simulink model "NonLinModelMracScaled"  (R2023b)
settings: Solver=ode4  StartTime=0.0  StopTime=50  FixedStep=1e-3  RelTol=1e-3
values from neighbouring files (symbols this model uses):
  Am_bar = A_bar - B_bar_mA * Km    [placePoles.m]
  B_bar_mA = B_bar .* 1e-3    [newDesign.m]
  Bm_bar_mm = B_bar_mA / DC_gain    [placePoles.m]
  Gamma_L = 1e-6    (= 1e-06)    [newDesign.m]
  Gamma_R = 1e-4    (= 0.0001)    [newDesign.m]
  L_hat_IC = -Km    [newDesign.m]
  M_hat_IC = 1 / DC_gain    [newDesign.m]
  P_bar = lyap(Am_bar', Q_bar)    [newDesign.m]
  P_return = 4.46e5    (= 446000)    [newDesign.m]
  PA_IC = PA_Pa.Data(1)    [newDesign.m]
  PB_IC = PB_Pa.Data(1)    [newDesign.m]
  Ps_supply = 199.85e5    (= 19985000)    [newDesign.m]
  sigma_L = 0.001    [newDesign.m]
  sigma_M = 0.001    [newDesign.m]
  xc_dot_IC = v_mPs.Data(1)    [newDesign.m]
  xc_IC = xc_m.Data(1)    [newDesign.m]
undefined symbols (not defined in the file or in its folder): AEFF, B_E, C_T, k, K, M, m3PsToLpm, PA_Pa, PB_Pa, r_v_mPs, V01, V02, V_DEAD, xc_m
settings Model: Creator=snr  LastModifiedBy=snr

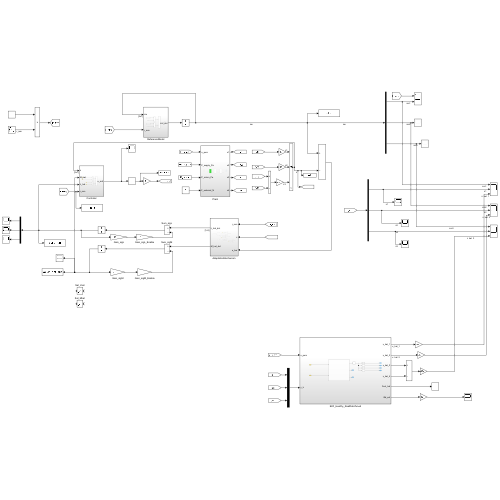
[thumbnail: Simulink's stored preview of the top-level diagram]
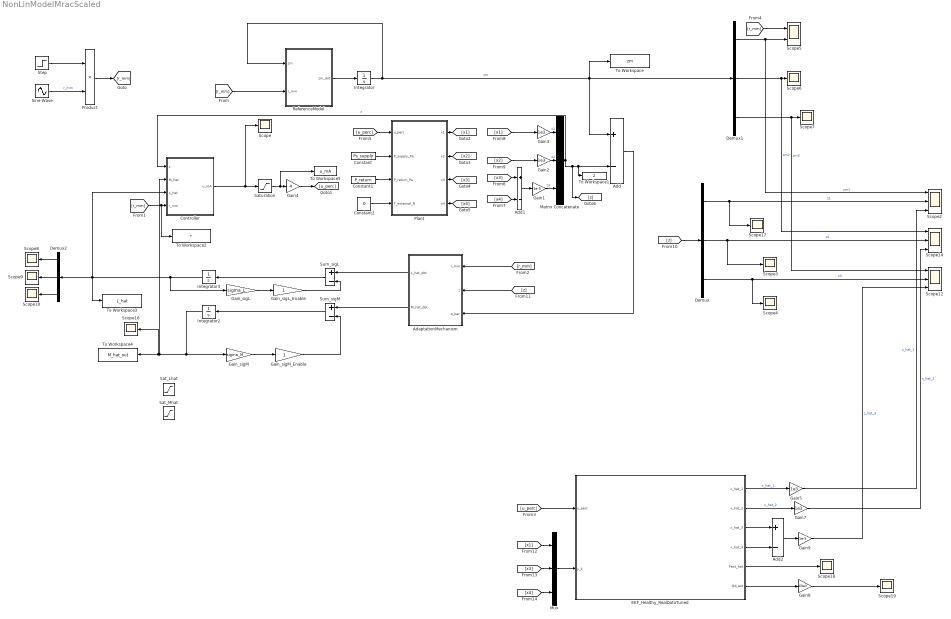
== system NonLinModelMracScaled ==
  AdaptationMechanism : Subsystem
  Add : Sum  Inputs=+-
  Add1 : Sum  Inputs=+-
  Add2 : Sum  Inputs=+-
  Constant : Constant  Value=Ps_supply
  Constant1 : Constant  Value=P_return
  Constant2 : Constant  Value=0
  Controller : Subsystem
  Demux : Demux  Outputs=3
  Demux1 : Demux  Outputs=3
  Demux2 : Demux  Outputs=3
  EKF_Healthy_RealDataTuned : Subsystem
  Gain1 : Gain  Gain=1e-5
  Gain{2..3,5,7} (4 alike) : Gain  Gain=1e3
  Gain4 : Gain  Gain=4
  Gain8 : Gain  Gain=60e3
  Gain9 : Gain  Gain=1e-5
  Gain_sigL : Gain  Gain=sigma_L
  Gain_sigL_Enable : Gain
  Gain_sigM : Gain  Gain=sigma_M
  Gain_sigM_Enable : Gain
  Integrator : Integrator  InitialCondition=[0;0;0]
  Integrator2 : Integrator  InitialCondition=M_hat_IC
  Integrator3 : Integrator  InitialCondition=L_hat_IC
  Matrix Concatenate : Concatenate  NumInputs=3  Mode=Multidimensional array
  Mux : Mux  Inputs=3
  Plant : Subsystem
  Product : Product
  ReferenceModel : Subsystem
  Sat_Lhat : Saturate  UpperLimit=0.125  LowerLimit=-0.125
  Sat_Mhat : Saturate  UpperLimit=0.12  LowerLimit=-0.12
  Saturation : Saturate  UpperLimit=25  LowerLimit=-25
  Scope{,3..4,6..10,16..19} (12 alike) : Scope
  Scope12 : Scope  NumInputPorts=3
  Scope14 : Scope  NumInputPorts=3
  Scope2 : Scope  NumInputPorts=3
  Scope5 : Scope  NumInputPorts=2
  Sine Wave : Sin  Amplitude=15  Frequency=2*pi*0.5  SampleTime=0
  Step : Step  Time=0  SampleTime=0
  Sum_sigL : Sum  Inputs=+-
  Sum_sigM : Sum  Inputs=+-
  To Workspace : ToWorkspace  VariableName=zm  SaveFormat=Timeseries  SampleTime=-1
  To Workspace1 : ToWorkspace  VariableName=z  SaveFormat=Timeseries  SampleTime=-1
  To Workspace2 : ToWorkspace  VariableName=r  SaveFormat=Timeseries  SampleTime=-1
  To Workspace3 : ToWorkspace  VariableName=L_hat  SaveFormat=Timeseries  SampleTime=-1
  To Workspace4 : ToWorkspace  VariableName=M_hat_out  SaveFormat=Timeseries  SampleTime=-1
  To Workspace5 : ToWorkspace  VariableName=u_mA  SaveFormat=Timeseries  SampleTime=-1
  wires:
  Constant2/1 -> Plant/4(F_external_N)
  Constant1/1 -> Plant/3(P_return_Pa)
  Gain1/1 -> Matrix Concatenate/3  "z3"
  Add1/1 -> Gain1/1
  Demux/2 -> Scope3/1, Scope14/2  "z2"
  Demux2/1 -> Scope8/1
  Demux2/3 -> Scope10/1
  [r_mm] -> ReferenceModel/2(r_mm)
  Demux2/2 -> Scope9/1
  Demux/3 -> Scope4/1, Scope12/2  "z3"
  [r_mm] -> AdaptationMechanism/1(r_mm)
  Sine Wave/1 -> Product/2  "r_mm"
  Demux1/1 -> Scope2/1, Scope5/2  "zm1"
  Demux1/2 -> Scope14/1, Scope6/1  "zm2"
  Integrator/1 -> To Workspace/1, Add/1, Demux1/1, ReferenceModel/1(zm)  "zm"
  Add/1 -> AdaptationMechanism/3(e_bar)
  Controller/1(u_mA) -> Scope/1, Saturation/1
  Demux1/3 -> Scope12/1, Scope7/1  "zm3"
  Demux/1 -> Scope17/1, Scope2/2  "z1"
  Constant/1 -> Plant/2(P_supply_Pa)
  Matrix Concatenate/1 -> [z], To Workspace1/1, Add/2, Controller/1(z)  "z"
  [r_mm] -> To Workspace2/1, Controller/4(r_mm)
  [r_mm] -> Scope5/1
  ReferenceModel/1(zm_dot) -> Integrator/1
  Gain2/1 -> Matrix Concatenate/2  "z2"
  Gain3/1 -> Matrix Concatenate/1  "z1"
  Saturation/1 -> To Workspace5/1, Gain4/1
  AdaptationMechanism/1(L_hat_dot) -> Sum_sigL/1
  Sum_sigL/1 -> Integrator3/1
  AdaptationMechanism/2(M_hat_dot) -> Sum_sigM/1
  Sum_sigM/1 -> Integrator2/1
  Step/1 -> Product/1
  Product/1 -> [r_mm]
  Mux/1 -> EKF_Healthy_RealDataTuned/2(y_k)
  EKF_Healthy_RealDataTuned/1(x_hat_1) -> Gain5/1  "x_hat_1"
  Gain5/1 -> Scope2/3  "z_hat_1"
  Gain4/1 -> [u_perc]
  EKF_Healthy_RealDataTuned/2(x_hat_2) -> Gain7/1  "x_hat_2"
  Gain7/1 -> Scope14/3  "z_hat_2"
  EKF_Healthy_RealDataTuned/5(Fext_hat) -> Scope18/1
  EKF_Healthy_RealDataTuned/6(Qd_est) -> Gain8/1
  Gain8/1 -> Scope19/1
  EKF_Healthy_RealDataTuned/4(x_hat_4) -> Add2/2
  EKF_Healthy_RealDataTuned/3(x_hat_3) -> Add2/1
  Add2/1 -> Gain9/1
  Gain9/1 -> Scope12/3  "z_hat_3"
  Integrator3/1 -> Gain_sigL/1, Demux2/1, To Workspace3/1, Controller/3(L_hat)
  Integrator2/1 -> Controller/2(M_hat), Scope16/1, To Workspace4/1, Gain_sigM/1
  Gain_sigM/1 -> Gain_sigM_Enable/1
  Gain_sigL/1 -> Gain_sigL_Enable/1
  Gain_sigM_Enable/1 -> Sum_sigM/2
  Gain_sigL_Enable/1 -> Sum_sigL/2
  [u_perc] -> EKF_Healthy_RealDataTuned/1(u_perc)
  [u_perc] -> Plant/1(u_perc)
  Plant/1(x1) -> [x1]
  Plant/2(x2) -> [x2]
  Plant/3(x3) -> [x3]
  Plant/4(x4) -> [x4]
  [x3] -> Add1/1
  [x4] -> Add1/2
  [x1] -> Gain3/1
  [x2] -> Gain2/1
  [z] -> Demux/1
  [z] -> AdaptationMechanism/2(z)
  [x1] -> Mux/1
  [x3] -> Mux/2
  [x4] -> Mux/3

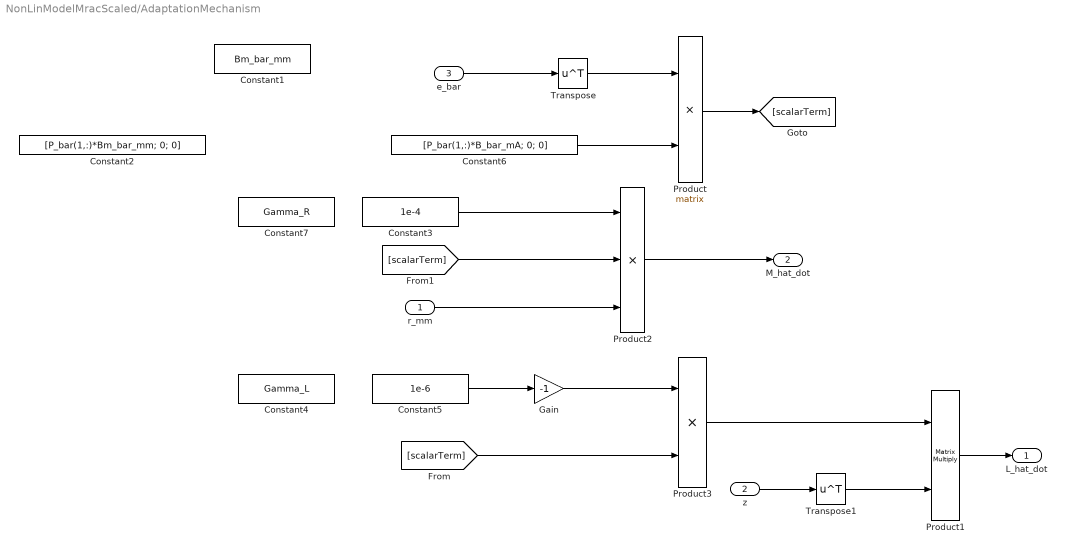
== system NonLinModelMracScaled/AdaptationMechanism ==
  r_mm : Inport
  z : Inport  Port=2
  e_bar : Inport  Port=3
  Constant1 : Constant  Value=Bm_bar_mm
  Constant2 : Constant  Value=[P_bar(1,:)*Bm_bar_mm; 0; 0]
  Constant3 : Constant  Value=1e-4
  Constant4 : Constant  Value=Gamma_L
  Constant5 : Constant  Value=1e-6
  Constant6 : Constant  Value=[P_bar(1,:)*B_bar_mA; 0; 0]
  Constant7 : Constant  Value=Gamma_R
  Gain : Gain  Gain=-1
  Product : Product  Multiplication=Matrix(*)
  Product1 : Product  Multiplication=Matrix(*)
  Product2 : Product  Inputs=3
  Product3 : Product
  Transpose : Math  Operator=transpose
  Transpose1 : Math  Operator=transpose
  L_hat_dot : Outport  PortDimensions=[1,3]
  M_hat_dot : Outport  Port=2
  wires:
  Gain/1 -> Product3/1
  Constant5/1 -> Gain/1
  Product1/1 -> L_hat_dot/1
  Transpose/1 -> Product/1
  Constant6/1 -> Product/2
  Product/1 -> [scalarTerm]
  [scalarTerm] -> Product3/2
  z/1 -> Transpose1/1
  Transpose1/1 -> Product1/2
  Product2/1 -> M_hat_dot/1
  Constant3/1 -> Product2/1
  [scalarTerm] -> Product2/2
  r_mm/1 -> Product2/3
  Product3/1 -> Product1/1
  e_bar/1 -> Transpose/1

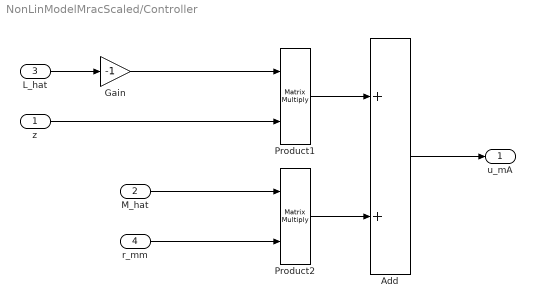
== system NonLinModelMracScaled/Controller ==
  z : Inport  PortDimensions=[3,1]
  M_hat : Inport  Port=2
  L_hat : Inport  Port=3
  r_mm : Inport  Port=4
  Add : Sum
  Gain : Gain  Gain=-1
  Product1 : Product  Multiplication=Matrix(*)
  Product2 : Product  Multiplication=Matrix(*)
  u_mA : Outport  PortDimensions=[1,1]
  wires:
  Add/1 -> u_mA/1
  Product1/1 -> Add/1
  Product2/1 -> Add/2
  L_hat/1 -> Gain/1
  z/1 -> Product1/2
  Gain/1 -> Product1/1
  M_hat/1 -> Product2/1
  r_mm/1 -> Product2/2

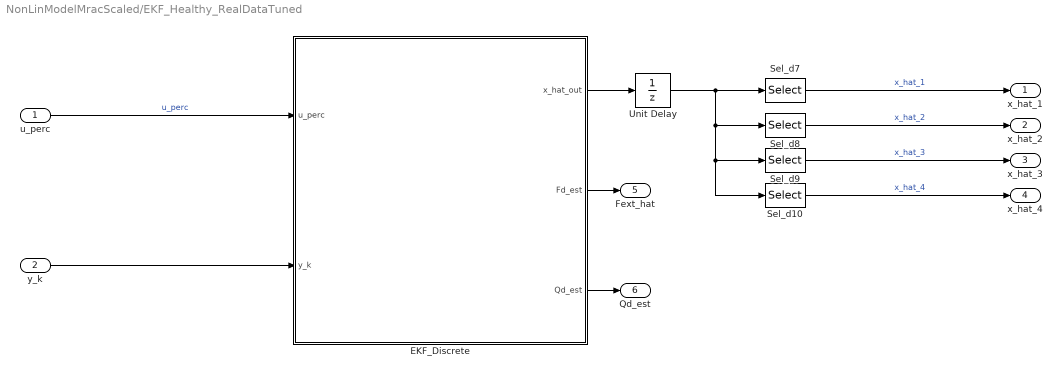
== system NonLinModelMracScaled/EKF_Healthy_RealDataTuned ==
  u_perc : Inport  OutDataTypeStr=double
  y_k : Inport  Port=2  OutDataTypeStr=double
  EKF_Discrete : MATLAB Function  TreatAsAtomicUnit=on  SystemSampleTime=1e-3
  Sel_d10 : Selector  InputPortWidth=6  IndexOptions=Index vector (dialog)  Indices=4  OutputSizes=1
  Sel_d7 : Selector  InputPortWidth=6  IndexOptions=Index vector (dialog)  Indices=1  OutputSizes=1
  Sel_d8 : Selector  InputPortWidth=6  IndexOptions=Index vector (dialog)  Indices=2  OutputSizes=1  RuntimeRangeChecks=on
  Sel_d9 : Selector  InputPortWidth=6  IndexOptions=Index vector (dialog)  Indices=3  OutputSizes=1
  Unit Delay : UnitDelay  InitialCondition=[xc_m.Data(1); r_v_mPs.Data(1); PA_Pa.Data(1); PB_Pa.Data(1); 0; 0]  SampleTime=1e-3  HasFrameUpgradeWarning=on
  x_hat_1 : Outport  OutDataTypeStr=double
  x_hat_2 : Outport  Port=2  OutDataTypeStr=double
  x_hat_3 : Outport  Port=3  OutDataTypeStr=double
  x_hat_4 : Outport  Port=4  OutDataTypeStr=double
  Fext_hat : Outport  Port=5  OutDataTypeStr=double
  Qd_est : Outport  Port=6  OutDataTypeStr=double
  wires:
  u_perc/1 -> EKF_Discrete/1(u_perc)  "u_perc"
  y_k/1 -> EKF_Discrete/2(y_k)
  EKF_Discrete/1(x_hat_out) -> Unit Delay/1
  Sel_d7/1 -> x_hat_1/1  "x_hat_1"
  Sel_d8/1 -> x_hat_2/1  "x_hat_2"
  Sel_d9/1 -> x_hat_3/1  "x_hat_3"
  Sel_d10/1 -> x_hat_4/1  "x_hat_4"
  EKF_Discrete/2(Fd_est) -> Fext_hat/1
  EKF_Discrete/3(Qd_est) -> Qd_est/1
  Unit Delay/1 -> Sel_d7/1, Sel_d10/1, Sel_d9/1, Sel_d8/1

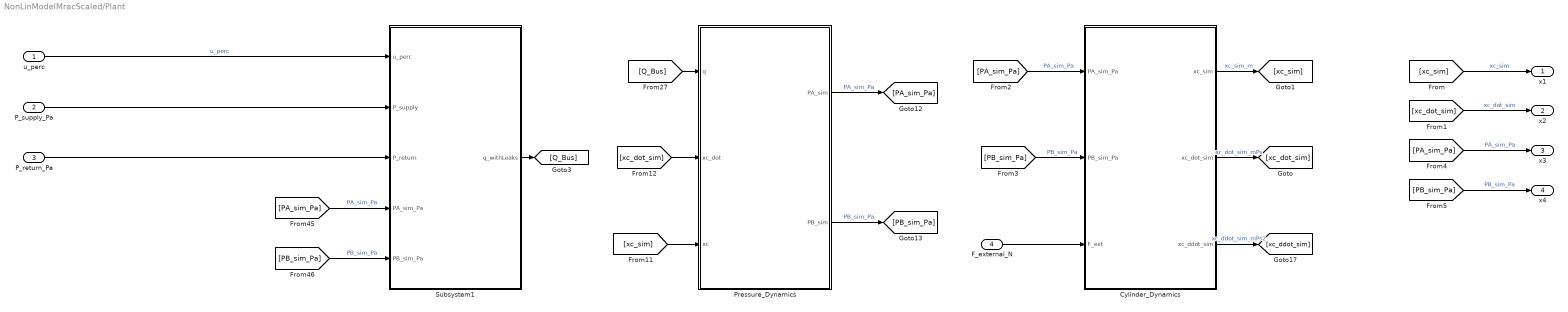
== system NonLinModelMracScaled/Plant ==
  u_perc : Inport  OutDataTypeStr=double
  P_supply_Pa : Inport  Port=2
  P_return_Pa : Inport  Port=3
  F_external_N : Inport  Port=4
  Cylinder_Dynamics : Subsystem
  Pressure_Dynamics : Subsystem
  Subsystem1 : Subsystem
  x1 : Outport
  x2 : Outport  Port=2
  x3 : Outport  Port=3
  x4 : Outport  Port=4
  wires:
  Cylinder_Dynamics/1(xc_sim) -> [xc_sim]  "xc_sim_m"
  [xc_sim] -> Pressure_Dynamics/3(xc)
  P_supply_Pa/1 -> Subsystem1/2(P_supply)
  [PA_sim_Pa] -> Subsystem1/4(PA_sim_Pa)  "PA_sim_Pa"
  [PB_sim_Pa] -> Subsystem1/5(PB_sim_Pa)  "PB_sim_Pa"
  [PB_sim_Pa] -> Cylinder_Dynamics/2(PB_sim_Pa)  "PB_sim_Pa"
  Pressure_Dynamics/1(PA_sim) -> [PA_sim_Pa]  "PA_sim_Pa"
  Cylinder_Dynamics/3(xc_ddot_sim) -> [xc_ddot_sim]  "xc_ddot_sim_mPs2"
  Cylinder_Dynamics/2(xc_dot_sim) -> [xc_dot_sim]  "xc_dot_sim_mPs"
  [xc_dot_sim] -> Pressure_Dynamics/2(xc_dot)
  [PA_sim_Pa] -> Cylinder_Dynamics/1(PA_sim_Pa)  "PA_sim_Pa"
  Pressure_Dynamics/2(PB_sim) -> [PB_sim_Pa]  "PB_sim_Pa"
  Subsystem1/1(q_withLeaks) -> [Q_Bus]
  [Q_Bus] -> Pressure_Dynamics/1(q)
  u_perc/1 -> Subsystem1/1(u_perc)  "u_perc"
  P_return_Pa/1 -> Subsystem1/3(P_return)
  F_external_N/1 -> Cylinder_Dynamics/3(F_ext)
  [xc_sim] -> x1/1  "xc_sim"
  [xc_dot_sim] -> x2/1  "xc_dot_sim"
  [PA_sim_Pa] -> x3/1  "PA_sim_Pa"
  [PB_sim_Pa] -> x4/1  "PB_sim_Pa"

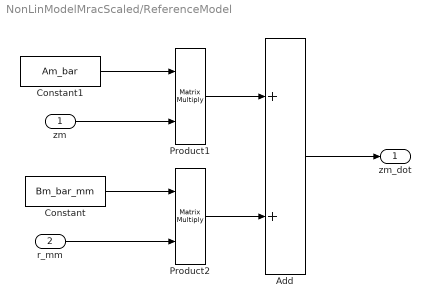
== system NonLinModelMracScaled/ReferenceModel ==
  zm : Inport  PortDimensions=[3,1]
  r_mm : Inport  Port=2  PortDimensions=[1,1]
  Add : Sum
  Constant : Constant  Value=Bm_bar_mm
  Constant1 : Constant  Value=Am_bar
  Product1 : Product  Multiplication=Matrix(*)
  Product2 : Product  Multiplication=Matrix(*)
  zm_dot : Outport
  wires:
  Constant/1 -> Product2/1
  Product2/1 -> Add/2
  r_mm/1 -> Product2/2
  Constant1/1 -> Product1/1
  zm/1 -> Product1/2
  Product1/1 -> Add/1
  Add/1 -> zm_dot/1

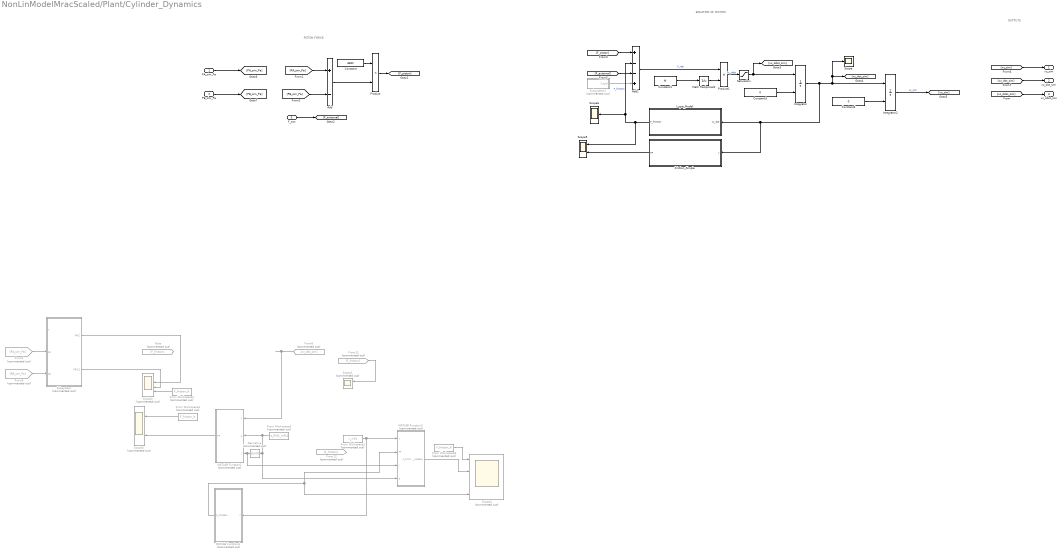
== system NonLinModelMracScaled/Plant/Cylinder_Dynamics ==
  note: PISTON FORCE
  note: EQUATION OF MOTION
  note: OUTPUTS
  PA_sim_Pa : Inport  OutDataTypeStr=double
  PB_sim_Pa : Inport  Port=2  OutDataTypeStr=double
  F_ext : Inport  Port=3  OutDataTypeStr=double
  Add : Sum  Inputs=+-
  Add1 : Sum  Inputs=+--+
  Constant : Constant  Value=AEFF  OutDataTypeStr=double
  Constant1 : Constant  Value=M  OutDataTypeStr=double
  Constant3 : Constant  Value=0
  Constant4 : Constant  Value=0
  Derivative : Derivative  Commented=on
  Friction_Simple : MATLAB Function  TreatAsAtomicUnit=on
  From Workspace1 : FromWorkspace  Commented=on  VariableName=v_mPs
  From Workspace2 : FromWorkspace  Commented=on  VariableName=F_friction_N
  From Workspace3 : FromWorkspace  Commented=on  VariableName=F_friction_N
  From Workspace4 : FromWorkspace  Commented=on  VariableName=F_friction_N
  From Workspace5 : FromWorkspace  Commented=on  VariableName=a_RMC_mPs2
  From11 : From  Commented=on  GotoTag=F_friction
  From12 : From  Commented=on  GotoTag=F_friction
  From4 : From  Commented=on  GotoTag=PA_sim_Pa
  From8 : From  Commented=on  GotoTag=xc_dot_sim
  From9 : From  Commented=on  GotoTag=PB_sim_Pa
  Goto : Goto  Commented=on  GotoTag=F_friction
  Integrator : Integrator  InitialConditionSource=external  InitialCondition=xc_dot_IC  UpperSaturationLimit=4  LowerSaturationLimit=-4
  Integrator2 : Integrator  InitialConditionSource=external  InitialCondition=xc_IC  LimitOutput=on  UpperSaturationLimit=0.09580  LowerSaturationLimit=-0.09580
  Lugre_Model : Subsystem
  MATLAB Function1 : MATLAB Function  Commented=on  TreatAsAtomicUnit=on
  MATLAB Function3 : MATLAB Function  Commented=on  TreatAsAtomicUnit=on
  MATLAB Function4 : MATLAB Function  Commented=on  TreatAsAtomicUnit=on
  Math Reciprocal2 : Math  Operator=reciprocal  SignedPower=on
  Product : Product
  Product1 : Product
  Saturation : Saturate  UpperLimit=100  LowerLimit=-100
  Scope : Scope
  Scope1 : Scope  Commented=on  NumInputPorts=2
  Scope2 : Scope  Commented=on  NumInputPorts=6
  Scope3 : Scope  Commented=on  NumInputPorts=2
  Scope4 : Scope  Commented=on  NumInputPorts=4
  Scope5 : Scope  NumInputPorts=2
  Scope6 : Scope
  Subsystem : Subsystem  Commented=on
  Subsystem1 : Subsystem  Commented=on
  xc_sim : Outport  OutDataTypeStr=double
  xc_dot_sim : Outport  Port=2  OutDataTypeStr=double
  xc_ddot_sim : Outport  Port=3  OutDataTypeStr=double
  wires:
  [PB_sim_Pa] -> Add/2
  [PA_sim_Pa] -> Add/1
  Add/1 -> Product/2
  Constant/1 -> Product/1
  Math Reciprocal2/1 -> Product1/2
  Product1/1 -> Saturation/1  "xc_ddot"
  Product/1 -> [F_piston]
  F_ext/1 -> [F_external]
  Add1/1 -> Product1/1  "F_net"
  Constant3/1 -> Integrator/2
  Integrator/1 -> Integrator2/1, Scope/1, [xc_dot_sim], Friction_Simple/1(v), Lugre_Model/1(xc_dot)
  Constant4/1 -> Integrator2/2
  Integrator2/1 -> [xc_sim]  "xc_sim"
  [xc_sim] -> xc_sim/1
  [xc_dot_sim] -> xc_dot_sim/1
  From8/1 -> MATLAB Function1/1(v)
  [xc_ddot_sim] -> xc_ddot_sim/1
  Saturation/1 -> [xc_ddot_sim], Integrator/1
  [F_external] -> Add1/3
  [F_piston] -> Add1/1
  ? -> Scope2/1, Goto/1  "F_friction"
  From Workspace2/1 -> Scope2/5
  Subsystem1/1(F_end) -> Add1/4
  PA_sim_Pa/1 -> [PA_sim_Pa]
  PB_sim_Pa/1 -> [PB_sim_Pa]
  From4/1 -> Subsystem/2(pa)
  From9/1 -> Subsystem/3(pb)
  Constant1/1 -> Math Reciprocal2/1
  Subsystem/2(FRIC1) -> Scope2/4
  Subsystem/1(FRIC) -> Scope2/3
  Derivative/1 -> MATLAB Function3/3(j), MATLAB Function1/3(j)
  From Workspace4/1 -> Scope3/1
  MATLAB Function1/1(FF) -> Scope3/2
  From Workspace5/1 -> MATLAB Function3/4(a), Derivative/1, MATLAB Function1/2(a)
  From11/1 -> Scope1/1
  From Workspace1/1 -> MATLAB Function4/1(v), MATLAB Function3/1(v)
  MATLAB Function3/1(F_friction_nodelay) -> Scope4/2
  From Workspace3/1 -> Scope4/1
  MATLAB Function4/1(F_stribeck) -> MATLAB Function3/2(FF), Scope4/4
  Lugre_Model/1(F_friction) -> Add1/2, Scope6/1, Scope5/1  "F_friction"
  Friction_Simple/1(FF) -> Scope5/2

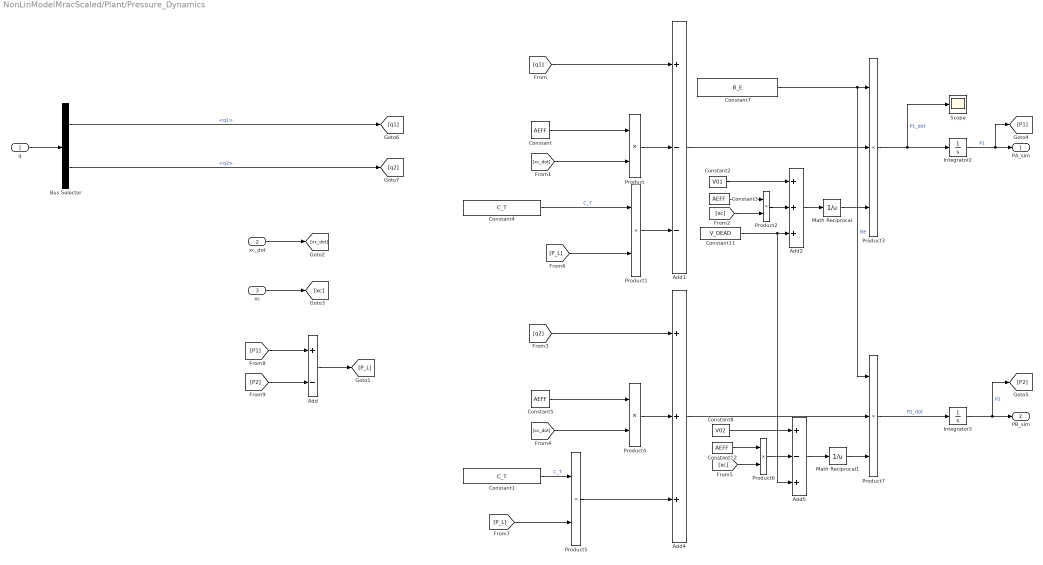
== system NonLinModelMracScaled/Plant/Pressure_Dynamics ==
  q : Inport  OutDataTypeStr=double
  xc_dot : Inport  Port=2  OutDataTypeStr=double
  xc : Inport  Port=3  OutDataTypeStr=double
  Add : Sum  Inputs=+-
  Add1 : Sum  Inputs=+--
  Add2 : Sum  Inputs=+++
  Add4 : Sum  Inputs=+++
  Add5 : Sum  Inputs=+-+
  Bus Selector : BusSelector  OutputSignals=q1,q2
  Constant{,3,5,12} (4 alike) : Constant  Value=AEFF  OutDataTypeStr=double
  Constant1 : Constant  Value=C_T  OutDataTypeStr=double
  Constant11 : Constant  Value=V_DEAD  OutDataTypeStr=double
  Constant2 : Constant  Value=V01  OutDataTypeStr=double
  Constant4 : Constant  Value=C_T  OutDataTypeStr=double
  Constant7 : Constant  Value=B_E  OutDataTypeStr=double
  Constant8 : Constant  Value=V02  OutDataTypeStr=double
  Integrator2 : Integrator  InitialCondition=PA_IC  LimitOutput=on  UpperSaturationLimit=200e5  LowerSaturationLimit=4e5
  Integrator3 : Integrator  InitialCondition=PB_IC  LimitOutput=on  UpperSaturationLimit=200e5  LowerSaturationLimit=4e5
  Math Reciprocal : Math  Operator=reciprocal  SignedPower=on
  Math Reciprocal1 : Math  Operator=reciprocal  SignedPower=on
  Product{,1..2,4..6} (6 alike) : Product
  Product3 : Product  Inputs=3
  Product7 : Product  Inputs=3
  Scope : Scope
  PA_sim : Outport  OutDataTypeStr=double
  PB_sim : Outport  Port=2  OutDataTypeStr=double
  wires:
  q/1 -> Bus Selector/1
  xc_dot/1 -> [xc_dot]
  [xc_dot] -> Product/2
  Constant/1 -> Product/1
  Integrator2/1 -> [P1], PA_sim/1  "P1"
  [P_L] -> Product1/2
  Product/1 -> Add1/2
  [q1] -> Add1/1
  xc/1 -> [xc]
  Constant2/1 -> Add2/1
  Product2/1 -> Add2/2
  [xc] -> Product2/2
  Constant3/1 -> Product2/1
  Add2/1 -> Math Reciprocal/1
  Product3/1 -> Integrator2/1, Scope/1  "P1_dot"
  Math Reciprocal/1 -> Product3/3
  Add1/1 -> Product3/2
  Constant7/1 -> Product7/1, Product3/1  "Be"
  Constant4/1 -> Product1/1  "C_T"
  [xc_dot] -> Product4/2
  Product4/1 -> Add4/2
  Add4/1 -> Product7/2
  Integrator3/1 -> [P2], PB_sim/1  "P2"
  [P_L] -> Product5/2
  Constant5/1 -> Product4/1
  Add5/1 -> Math Reciprocal1/1
  [q2] -> Add4/1
  Math Reciprocal1/1 -> Product7/3
  Product7/1 -> Integrator3/1  "P2_dot"
  [xc] -> Product6/2
  Constant8/1 -> Add5/1
  Constant12/1 -> Product6/1
  Product6/1 -> Add5/2
  Bus Selector/2 -> [q2]  "<q2>"
  Bus Selector/1 -> [q1]  "<q1>"
  [P2] -> Add/2
  [P1] -> Add/1
  Add/1 -> [P_L]
  Constant1/1 -> Product5/1  "C_T"
  Product5/1 -> Add4/3
  Product1/1 -> Add1/3
  Constant11/1 -> Add5/3, Add2/3

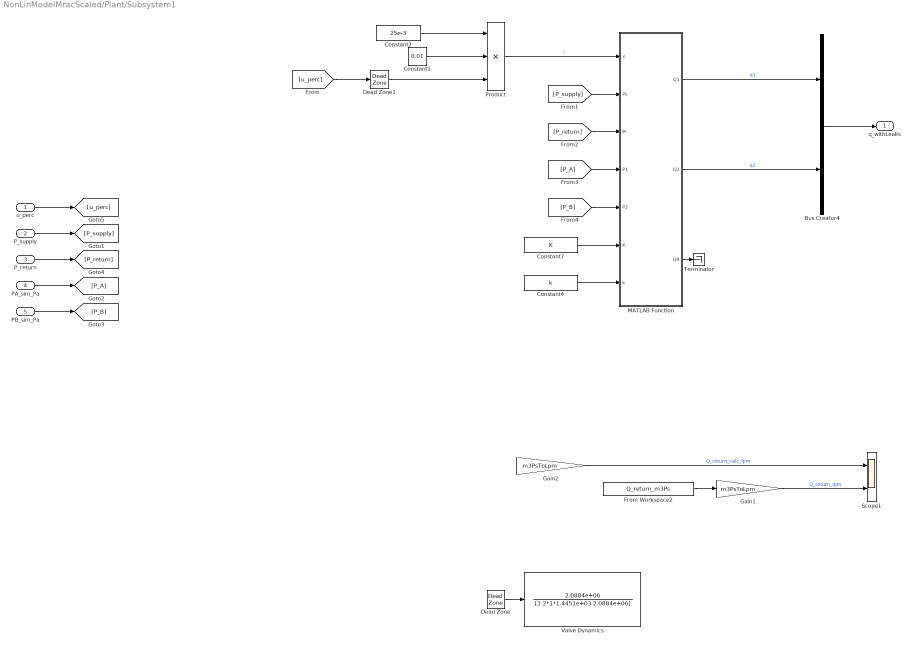
== system NonLinModelMracScaled/Plant/Subsystem1 ==
  u_perc : Inport  OutDataTypeStr=double
  P_supply : Inport  Port=2  OutDataTypeStr=double
  P_return : Inport  Port=3  OutDataTypeStr=double
  PA_sim_Pa : Inport  Port=4  OutDataTypeStr=double
  PB_sim_Pa : Inport  Port=5  OutDataTypeStr=double
  Bus Creator4 : BusCreator  Inputs=2
  Constant1 : Constant  Value=0.01
  Constant2 : Constant  Value=25e-3
  Constant4 : Constant  Value=k
  Constant7 : Constant  Value=K
  Dead Zone : DeadZone  LowerValue=-0.02  UpperValue=0.02
  Dead Zone1 : DeadZone  LowerValue=-0.02  UpperValue=0.02
  From Workspace2 : FromWorkspace  VariableName=Q_return_m3Ps
  Gain1 : Gain  Gain=m3PsToLpm
  Gain2 : Gain  Gain=m3PsToLpm
  MATLAB Function : MATLAB Function  TreatAsAtomicUnit=on
  Product : Product  Inputs=3
  Scope1 : Scope  NumInputPorts=2
  Terminator : Terminator
  Valve Dynamics : TransferFcn  Numerator=[2.0884e+06]  Denominator=[1 2*1*1.4451e+03 2.0884e+06]
  q_withLeaks : Outport  OutDataTypeStr=double
  wires:
  PA_sim_Pa/1 -> [P_A]
  P_supply/1 -> [P_supply]
  P_return/1 -> [P_return]
  PB_sim_Pa/1 -> [P_B]
  u_perc/1 -> [u_perc]
  [P_supply] -> MATLAB Function/2(Ps)
  [P_return] -> MATLAB Function/3(Pr)
  [P_A] -> MATLAB Function/4(P1)
  [P_B] -> MATLAB Function/5(P2)
  Bus Creator4/1 -> q_withLeaks/1
  MATLAB Function/1(Q1) -> Bus Creator4/1  "q1"
  MATLAB Function/2(Q2) -> Bus Creator4/2  "q2"
  Constant2/1 -> Product/1
  Product/1 -> MATLAB Function/1(x)  "i"
  Constant1/1 -> Product/2
  Constant4/1 -> MATLAB Function/7(k)
  Constant7/1 -> MATLAB Function/6(K)
  [u_perc] -> Dead Zone1/1
  From Workspace2/1 -> Gain1/1
  Gain2/1 -> Scope1/1  "Q_return_calc_lpm"
  Gain1/1 -> Scope1/2  "Q_return_lpm"
  MATLAB Function/3(QR) -> Terminator/1
  Dead Zone/1 -> Valve Dynamics/1
  Dead Zone1/1 -> Product/3

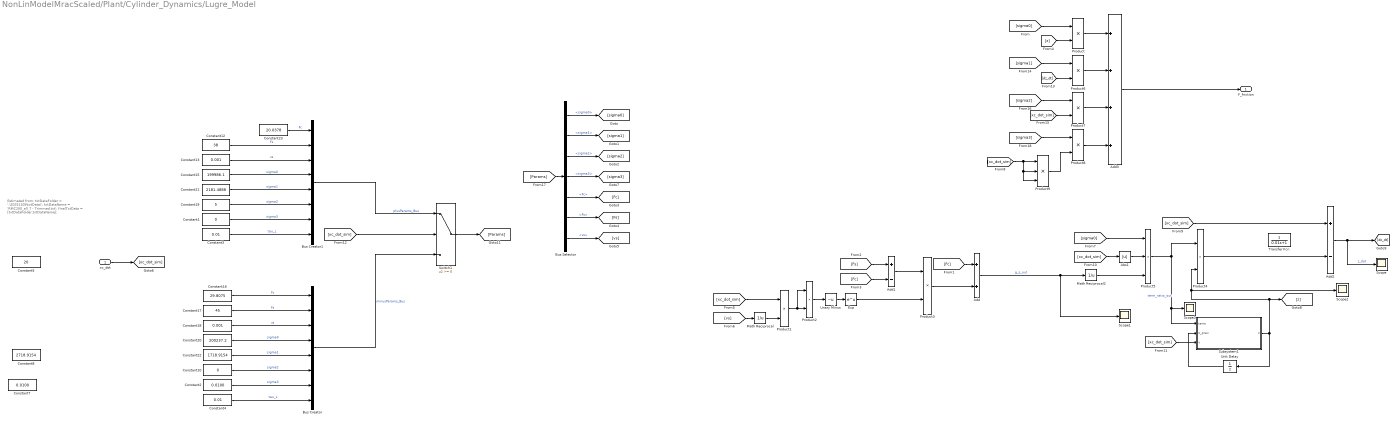
== system NonLinModelMracScaled/Plant/Cylinder_Dynamics/Lugre_Model ==
  note: Estimated from:
      |
      | txtDataFolder = '.\20251105\txtData\';
      | txtDataName = 'RMC200_all_7 - Trimmed.txt';
      | finalTxtData = [txtDataFolder,txtDataName];
  xc_dot : Inport  OutDataTypeStr=double
  Abs1 : Abs  SaturateOnIntegerOverflow=off
  Add : Sum
  Add1 : Sum  Inputs=+-
  Add2 : Sum  Inputs=+-
  Add3 : Sum  Inputs=++++
  Bus Selector : BusSelector  OutputSignals=sigma0,sigma1,sigma2,sigma3,Fc,Fs,vs
  Bus Creator : BusCreator  Inputs=8
  Bus Creator1 : BusCreator  Inputs=8
  Constant1 : Constant  Value=0  OutDataTypeStr=double
  Constant10 : Constant  Value=0  OutDataTypeStr=double
  Constant12 : Constant  Value=38  OutDataTypeStr=double
  Constant13 : Constant  Value=0.001  OutDataTypeStr=double
  Constant15 : Constant  Value=199986.1  OutDataTypeStr=double
  Constant16 : Constant  Value=29.8075  OutDataTypeStr=double
  Constant17 : Constant  Value=45  OutDataTypeStr=double
  Constant18 : Constant  Value=0.001  OutDataTypeStr=double
  Constant19 : Constant  Value=5  OutDataTypeStr=double
  Constant2 : Constant  Value=0.0100  OutDataTypeStr=double
  Constant20 : Constant  Value=200237.2  OutDataTypeStr=double
  Constant21 : Constant  Value=2181.4888  OutDataTypeStr=double
  Constant22 : Constant  Value=1718.9154  OutDataTypeStr=double
  Constant23 : Constant  Value=20.0378  OutDataTypeStr=double
  Constant3 : Constant  Value=0.01  OutDataTypeStr=double
  Constant4 : Constant  Value=0.01  OutDataTypeStr=double
  Constant5 : Constant  Value=20  OutDataTypeStr=double
  Constant7 : Constant  Value=0.0100  OutDataTypeStr=double
  Constant8 : Constant  Value=2718.9154  OutDataTypeStr=double
  Exp : Math  SignedPower=on
  Math Reciprocal : Math  Operator=reciprocal  SignedPower=on
  Math Reciprocal2 : Math  Operator=reciprocal  SignedPower=on
  Product{,1..4,6..8} (8 alike) : Product
  Product5 : Product  Inputs=3
  Product9 : Product  Inputs=3
  Scope{,1..3} (4 alike) : Scope
  Subsystem1 : Subsystem
  Switch1 : Switch  SaturateOnIntegerOverflow=off  InputSameDT=off
  Transfer Fcn : TransferFcn  Denominator=[0.01 1]
  Unary Minus : UnaryMinus
  Unit Delay : UnitDelay  SampleTime=-1  HasFrameUpgradeWarning=on
  F_friction : Outport
  wires:
  Constant18/1 -> Bus Creator/3  "vs"
  Constant13/1 -> Bus Creator1/3  "vs"
  Constant12/1 -> Bus Creator1/2  "Fs"
  Constant17/1 -> Bus Creator/2  "Fs"
  Constant22/1 -> Bus Creator/5  "sigma1"
  Constant20/1 -> Bus Creator/4  "sigma0"
  Constant10/1 -> Bus Creator/6  "sigma2"
  Constant16/1 -> Bus Creator/1  "Fc"
  Constant21/1 -> Bus Creator1/5  "sigma1"
  Constant15/1 -> Bus Creator1/4  "sigma0"
  Constant19/1 -> Bus Creator1/6  "sigma2"
  Product7/1 -> Add3/3
  Product6/1 -> Add3/2
  [sigma2] -> Product7/1
  [xc_dot_sim] -> Product7/2
  [dz_dt] -> Product6/2
  [sigma1] -> Product6/1
  Product/1 -> Add3/1
  [z] -> Product/2
  [sigma0] -> Product5/1
  Abs1/1 -> Product5/2
  Add/1 -> Math Reciprocal2/1, Scope1/1  "g_s_out"
  [xc_dot_sim] -> Abs1/1
  Add1/1 -> Product3/1
  Unary Minus/1 -> Exp/1
  Product2/1 -> Unary Minus/1
  Product1/1 -> Product2/2, Product2/1
  [xc_dot_sim] -> Product1/1
  Math Reciprocal/1 -> Product1/2
  [vs] -> Math Reciprocal/1
  [Fc] -> Add1/2
  [Fs] -> Add1/1
  [Fc] -> Add/1
  [sigma0] -> Product/1
  Product3/1 -> Add/2
  Bus Creator1/1 -> Switch1/1  "plusParams_Bus"
  Bus Creator/1 -> Switch1/3  "minusParams_Bus"
  [Params] -> Bus Selector/1
  Bus Selector/1 -> [sigma0]  "<sigma0>"
  Bus Selector/2 -> [sigma1]  "<sigma1>"
  Bus Selector/3 -> [sigma2]  "<sigma2>"
  Bus Selector/5 -> [Fc]  "<Fc>"
  Bus Selector/6 -> [Fs]  "<Fs>"
  Bus Selector/7 -> [vs]  "<vs>"
  Math Reciprocal2/1 -> Product5/3
  Exp/1 -> Product3/2
  Add2/1 -> Scope/1, [dz_dt]  "z_dot"
  [xc_dot_sim] -> Switch1/2
  [xc_dot_sim] -> Add2/1
  [xc_dot_sim] -> Subsystem1/3(v)
  Unit Delay/1 -> Subsystem1/2(z_prev)
  Product5/1 -> Scope3/1, Subsystem1/1(term), Product4/1  "term_ratio_out"
  Add3/1 -> F_friction/1
  Constant1/1 -> Bus Creator1/7  "sigma3"
  Constant2/1 -> Bus Creator/7  "sigma3"
  Constant3/1 -> Bus Creator1/8  "tau_L"
  Constant4/1 -> Bus Creator/8  "tau_L"
  [sigma3] -> Product8/1
  Product8/1 -> Add3/4
  [xc_dot_sim] -> Product9/2, Product9/3, Product9/1
  Product9/1 -> Product8/2
  Bus Selector/4 -> [sigma3]  "<sigma3>"
  xc_dot/1 -> [xc_dot_sim]
  Constant23/1 -> Bus Creator1/1  "Fc"
  Subsystem1/1(z) -> Scope2/1, Product4/2, [z], Unit Delay/1
  Switch1/1 -> [Params]
  Product4/1 -> Add2/2

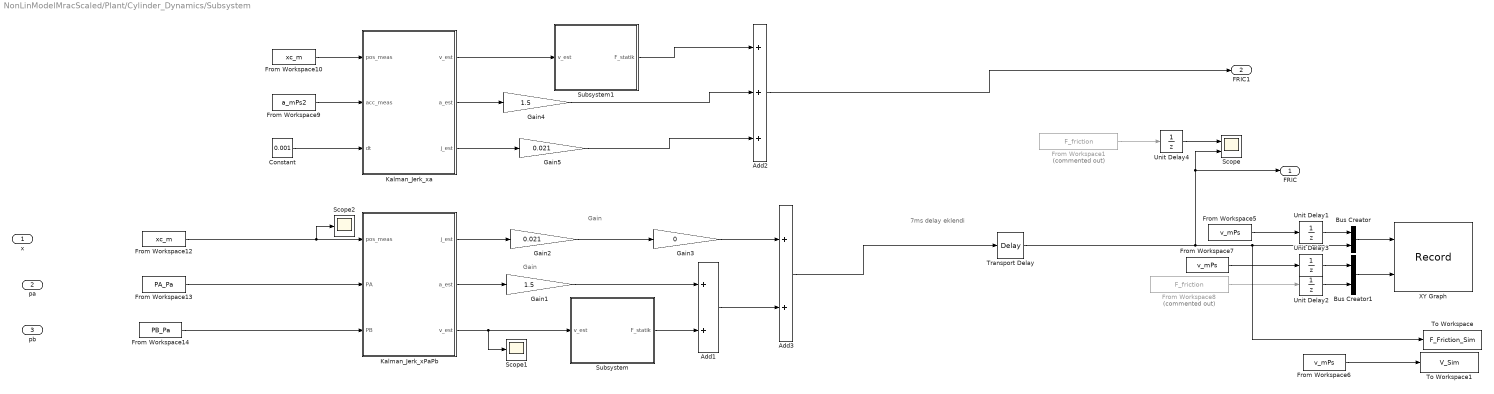
== system NonLinModelMracScaled/Plant/Cylinder_Dynamics/Subsystem ==
  note: Gain
  note: 7ms delay eklendi
  note: Gain
  x : Inport
  pa : Inport  Port=2
  pb : Inport  Port=3
  Add1 : Sum
  Add2 : Sum  Inputs=+++
  Add3 : Sum
  Bus Creator : BusCreator  Inputs=2
  Bus Creator1 : BusCreator  Inputs=2
  Constant : Constant  Value=0.001
  From Workspace1 : FromWorkspace  Commented=on  VariableName=F_friction
  From Workspace10 : FromWorkspace  VariableName=xc_m
  From Workspace12 : FromWorkspace  VariableName=xc_m
  From Workspace13 : FromWorkspace  VariableName=PA_Pa
  From Workspace14 : FromWorkspace  VariableName=PB_Pa
  From Workspace5 : FromWorkspace  VariableName=v_mPs
  From Workspace6 : FromWorkspace  VariableName=v_mPs
  From Workspace7 : FromWorkspace  VariableName=v_mPs
  From Workspace8 : FromWorkspace  Commented=on  VariableName=F_friction
  From Workspace9 : FromWorkspace  VariableName=a_mPs2
  Gain1 : Gain  Gain=1.5
  Gain2 : Gain  Gain=0.021
  Gain3 : Gain  Gain=0
  Gain4 : Gain  Gain=1.5
  Gain5 : Gain  Gain=0.021
  Kalman_Jerk_xPaPb : MATLAB Function  TreatAsAtomicUnit=on
  Kalman_Jerk_xa : MATLAB Function  TreatAsAtomicUnit=on
  Scope : Scope  NumInputPorts=2
  Scope1 : Scope
  Scope2 : Scope
  Subsystem : Subsystem
  Subsystem1 : Subsystem
  To Workspace : ToWorkspace  VariableName=F_Friction_Sim  SaveFormat=Timeseries  SampleTime=-1
  To Workspace1 : ToWorkspace  VariableName=V_Sim  SaveFormat=Timeseries  SampleTime=-1
  Transport Delay : TransportDelay  DelayTime=7e-3
  Unit Delay{1..4} (4 alike) : UnitDelay  SampleTime=-1  HasFrameUpgradeWarning=on
  XY Graph : Record  FileSettingsInternal="{\"entries\":[{\"content\":{\"excelSettings\":{\"content\":{},\"type\":\"Streamout.ExcelSettings\"}},\"type\":\"Streamout.FileSettingStorage\",\"uuid\":\"\"}],\"packageUris\":[\"http:\\/\\/schema.mathworks.com\\/mf0\\/streamout_blocks\\/R2020a\"],\"version\":\"1.0\"}"  Layout=[1 1]  SignalsInternal="{\"entries\":[{\"content\":{},\"type\":\"RecordBlkView.InputSignals\",\"uuid\":\"\"}],\"packageUris\":[\"http:\\/\\/schema.mathworks.com\\/mf0\\/streamout_blocks\\/R2020a\"],\"version\":\"1.0\"}"  VisualizationBindings="{\"xyplotplugin\":{\"info\":[{\"series\":[],\"subplotID\":1}]}}"  CompatibilityTag=XY
  FRIC : Outport
  FRIC1 : Outport  Port=2
  wires:
  Unit Delay2/1 -> Bus Creator1/2
  From Workspace9/1 -> Kalman_Jerk_xa/2(acc_meas)
  Constant/1 -> Kalman_Jerk_xa/3(dt)
  From Workspace12/1 -> Scope2/1, Kalman_Jerk_xPaPb/1(pos_meas)
  From Workspace7/1 -> Unit Delay3/1
  Unit Delay3/1 -> Bus Creator1/1
  From Workspace13/1 -> Kalman_Jerk_xPaPb/2(PA)
  Add3/1 -> Transport Delay/1
  Bus Creator1/1 -> XY Graph/2
  From Workspace10/1 -> Kalman_Jerk_xa/1(pos_meas)
  From Workspace5/1 -> Unit Delay1/1
  Bus Creator/1 -> XY Graph/1
  From Workspace14/1 -> Kalman_Jerk_xPaPb/3(PB)
  Kalman_Jerk_xPaPb/1(j_est) -> Gain2/1
  From Workspace8/1 -> Unit Delay2/1
  Kalman_Jerk_xPaPb/2(a_est) -> Gain1/1
  From Workspace6/1 -> To Workspace1/1
  Unit Delay1/1 -> Bus Creator/1
  Kalman_Jerk_xPaPb/3(v_est) -> Scope1/1, Subsystem/1(v_est)
  From Workspace1/1 -> Unit Delay4/1
  Unit Delay4/1 -> Scope/1
  Transport Delay/1 -> Scope/2, FRIC/1, Bus Creator/2, To Workspace/1
  Subsystem/1(F_statik) -> Add1/2
  Gain1/1 -> Add1/1
  Gain2/1 -> Gain3/1
  Add1/1 -> Add3/2
  Gain3/1 -> Add3/1
  Kalman_Jerk_xa/2(a_est) -> Gain4/1
  Kalman_Jerk_xa/1(v_est) -> Subsystem1/1(v_est)
  Subsystem1/1(F_statik) -> Add2/1
  Gain4/1 -> Add2/2
  Add2/1 -> FRIC1/1
  Kalman_Jerk_xa/3(j_est) -> Gain5/1
  Gain5/1 -> Add2/3

== system NonLinModelMracScaled/Plant/Cylinder_Dynamics/Subsystem1 ==
  Constant2 : Constant  Value=-0.09580
  Constant5 : Constant  Value=0.09580
  Constant6 : Constant  Value=1e6
  Constant7 : Constant  Value=2e-3
  MATLAB Function1 : MATLAB Function  TreatAsAtomicUnit=on
  F_end : Outport
  wires:
  Constant7/1 -> MATLAB Function1/6(v_lock)
  [xc_sim] -> MATLAB Function1/1(x)
  [xc_dot_sim] -> MATLAB Function1/2(x_dot)
  Constant6/1 -> MATLAB Function1/5(k_end)
  Constant2/1 -> MATLAB Function1/3(xmin)
  Constant5/1 -> MATLAB Function1/4(xmax)
  MATLAB Function1/1(F_end) -> F_end/1

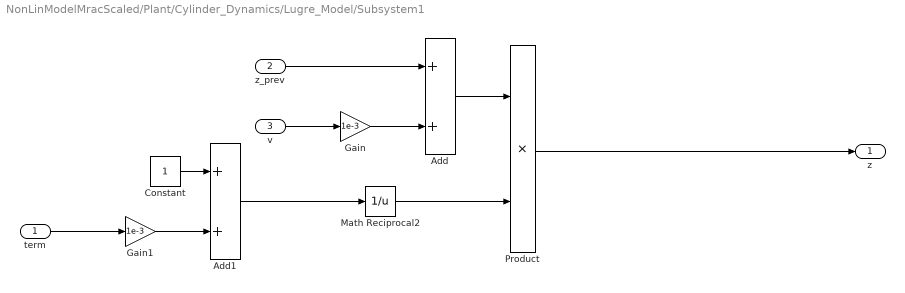
== system NonLinModelMracScaled/Plant/Cylinder_Dynamics/Lugre_Model/Subsystem1 ==
  term : Inport
  z_prev : Inport  Port=2
  v : Inport  Port=3
  Add : Sum
  Add1 : Sum
  Constant : Constant
  Gain : Gain  Gain=1e-3
  Gain1 : Gain  Gain=1e-3
  Math Reciprocal2 : Math  Operator=reciprocal  SignedPower=on
  Product : Product
  z : Outport
  wires:
  term/1 -> Gain1/1
  z_prev/1 -> Add/1
  v/1 -> Gain/1
  Gain/1 -> Add/2
  Add/1 -> Product/1
  Gain1/1 -> Add1/2
  Constant/1 -> Add1/1
  Add1/1 -> Math Reciprocal2/1
  Math Reciprocal2/1 -> Product/2
  Product/1 -> z/1

== system NonLinModelMracScaled/Plant/Cylinder_Dynamics/Subsystem/Subsystem ==
  v_est : Inport
  MATLAB Function : MATLAB Function  TreatAsAtomicUnit=on
  F_statik : Outport
  wires:
  v_est/1 -> MATLAB Function/1(v)
  MATLAB Function/1(F_statik) -> F_statik/1

== system NonLinModelMracScaled/Plant/Cylinder_Dynamics/Subsystem/Subsystem1 ==
  v_est : Inport
  MATLAB Function : MATLAB Function  TreatAsAtomicUnit=on
  F_statik : Outport
  wires:
  MATLAB Function/1(F_statik) -> F_statik/1
  v_est/1 -> MATLAB Function/1(v)

== matlab function NonLinModelMracScaled/Plant/Cylinder_Dynamics/MATLAB Function3 ==
  data: v input; F_friction_nodelay output; FF input; j input; a input
function F_friction_nodelay = fcn(v, FF, j, a)

K_acc_p = 1.021235; 
K_acc_n = 0.0810121235; 

K_jerk_p = -0.05656481; 
K_jerk_n = 0.02056481; 

K_acc = (v>=0)*K_acc_p + (v<0)*K_acc_n; 
K_jerk = (v>=0)*K_jerk_p + (v<0)*K_jerk_n; 

F_friction_nodelay = FF + K_acc .* a  +  K_jerk.*j;

== matlab function NonLinModelMracScaled/Plant/Cylinder_Dynamics/MATLAB Function4 ==
  data: v input; F_stribeck output
function F_stribeck = fcn(v)


% close all 

% --- Geçiş Yumuşaklığı Parametresi ---
% Bu değer büyüdükçe 0'daki eğim azalır (daha eğimli geçer)
eps_smooth = 0.0223;
% eps_smooth = 0.015;

%%%
kv_p = 12; Fc_p = 25; Fs_p  = 383; tau_p = 0.016;
kv_n = 35; Fc_n = 7.5; Fs_n = 183; tau_n = 0.02016;
%%%


% Yumuşatılmış yön fonksiyonu (sign yerine tanh)
% Bu fonksiyon -1 ile 1 arasında yumuşak bir geçiş sağlar
smooth_sign = tanh(v ./ eps_smooth);

% Asimetrik katsayı vektörleri oluşturma
% Hızın yönüne göre katsayıları seçiyoruz
kv = (v >= 0)*kv_p + (v < 0)*kv_n;
Fc = (v >= 0)*Fc_p + (v < 0)*Fc_n;
Fs = (v >= 0)*Fs_p + (v < 0)*Fs_n;
tau = (v >= 0)*tau_p + (v < 0)*tau_n;
F_stribeck = (kv .* v) + (Fc .* smooth_sign) + (Fs .* smooth_sign .* exp(-abs(v./tau)));

== matlab function NonLinModelMracScaled/EKF_Healthy_RealDataTuned/EKF_Discrete ==
  data: u_perc input; x_hat_out output; y_k input; Fd_est output; Qd_est output
function [x_hat_out, Fd_est, Qd_est] = sdre_6state_crio(u_perc, y_k)
%SDRE_6STATE_CRIO  Discrete 6-state Extended State Observer (ESO)
%  Fully Physical Formulation: A(x) contains internal dynamics.
%  f(x,u) contains physical flows and hard friction nonlinearities.
%  Includes x5 (Mismatched Mech Disturbance) and x6 (Matched Hyd Disturbance).
%
%  States:  x = [pos(m), vel(m/s), PA(Pa), PB(Pa), Fd(N), Qd(m^3/s)]
%  Inputs:  u_k   - valve spool displacement command [m] (max 25e-5)
%           y_k   - [pos_m; PA_Pa; PB_Pa]  (measurements)
%           Ps_k  - supply pressure [Pa]
%           Pr_k  - return pressure [Pa]
%  Outputs: x_hat_out - [pos; vel; PA; PB; Fd; Qd] state estimate
%           Fd_est    - Estimated mechanical load/friction mismatch [N]
%           Qd_est    - Estimated hydraulic internal leakage/valve mismatch [m^3/s]
%#codegen

%% ── PERSISTENT STATE ─────────────────────────────────────────────────────
persistent x_hat P_k initialized;

%% ── SYSTEM PARAMETERS ────────────────────────────────────────────────────
M       = 3.4;
d_p     = 34e-3;   
d_r     = 30e-3;
A_c     = pi/4*(d_p^2 - d_r^2);   
V_dead  = 1.5315e-5;
V_0     = A_c*(190.16e-3/2) + V_dead;   
C_t     = 3.9933e-13;
beta    = 1.6e9;
Ps_k    = 200e5; 
Pr_k    = 4e5; 

% Valve Parameters
K_sv    = 3.34e-6;
k_sv    = 1.82709080;
x0_S    = 0.46e-3;
x0_R    = 0.64e-3;
K_tare  = 2.345e-9; 
u_k     = u_perc * 25e-5; % Scale % to 25mA
% Observer design
dt          = 1e-3;
alpha_Fd    = 1e-2;   % Mechanical disturbance decay factor
alpha_Qd    = 0.2;    % Hydraulic disturbance decay factor

% Tuning Matrices (Optimized for robust model-measurement balance)
% Q_d6 = diag([1E-12,... %x1
%              1E-5,... %x2
%              1E0, 1E0, ... %x3 x4
%              1E-7, ... %Fd
%              1e-3]); %Qd

% Q_d6: x5 serbest bırakıldı, x2 esnetildi
% Q_d6: Kinematiği katılaştırıp, x5'i öğrenmeye açıyoruz
Q_d6 = diag([1E-14, ... % x1: dx1/dt = x2 ilişkisi KUSURSUZ kabul edilsin (Titremeyi bu önler)
             5E-5,  ... % x2: Hızın tepe noktalarına çıkış izni
             1E0,   ... % x3: PA
             1E0,   ... % x4: PB
             1E-2,  ... % x5: Fd_est ÇOK hızlı güncellensin (Asimetrik sürtünmeyi anında öğrensin)
             1E-3]);... % x6: Qd_est

% Tuning Matrices (Optimized for robust model-measurement balance)
% Q_d6 = diag([1E-12,... %x1
%              1E-6,... %x2
%              1E0, 1E0, ... %x3 x4
%              1E-3, ... %Fd
%              1e-3]); %Qd

R_m6 = diag([1E-10, 5E-2, 5E-2]);

% Scaling (Qd is ~1e-5 m^3/s, so we scale by 1e5 to keep it ~1.0)
SC6  = [1; 1; 1e-7; 1e-7; 1e-2; 1e5];
SCI6 = [1; 1; 1e7;  1e7;  1e2;  1e-5]; % <--- Son eleman 1e-5 OLMAK ZORUNDA
I6   = eye(6);
C_sc6 = [1 0 0 0 0 0; 
         0 0 1 0 0 0; 
         0 0 0 1 0 0];

%% ── INITIALIZATION ───────────────────────────────────────────────────────
if isempty(initialized)
    % Initialize 6 states
    x_hat = [y_k(1); 0; y_k(2); y_k(3); 0; 0];
    P_k   = diag([1e-6, 1e-4, 1e-6, 1e-6, 1e-4, 1e-6]);
    initialized = true;
end

%% ── STATE EXTRACTION ────────────────────────────────────────────────────
x1 = x_hat(1); % Position
x2 = x_hat(2); % Velocity
x3 = x_hat(3); % PA
x4 = x_hat(4); % PB

%% ── STEP 1: Asymmetric Friction (Linear/Nonlinear Split) ────────────────
kv = 38;

% % A6 Matrix component (Linear Viscous Damping)
a22 = -kv / M;

F_nl = 0;



%% ── STEP 2: Robust Physical Valve Flows ─────────────────────────────────
% P_tol prevents zero derivative (inf gain) when pressure hits rails
P_tol = 0.1*1e5; % 0.1 bar tolerance


PA_c = max(Pr_k + P_tol, min(Ps_k - P_tol, x3));
PB_c = max(Pr_k + P_tol, min(Ps_k - P_tol, x4));

if u_k >= 0
    Q1_s = K_sv * sqrt(Ps_k - PA_c) * (x0_S + u_k);
    Q1_r = K_sv * sqrt(PA_c - Pr_k) * (x0_R^2 / (x0_R + k_sv*u_k));
    
    Q2_s = K_sv * sqrt(Ps_k - PB_c) * (x0_S^2 / (x0_S + k_sv*u_k)); 
    Q2_r = K_sv * sqrt(PB_c - Pr_k) * (x0_R + u_k);
else
    Q1_s = K_sv * sqrt(Ps_k - PA_c) * (x0_S^2 / (x0_S - k_sv*u_k));
    Q1_r = K_sv * sqrt(PA_c - Pr_k) * (x0_R - u_k);
    
    Q2_s = K_sv * sqrt(Ps_k - PB_c) * (x0_S - u_k);
    Q2_r = K_sv * sqrt(PB_c - Pr_k) * (x0_R^2 / (x0_R - k_sv*u_k));
end

Q1 = Q1_s - Q1_r; % Net flow into A
Q2 = Q2_s - Q2_r; % Net flow into B
% Q_return = Q1_R + Q2_R + K_tare * sqrt(Ps_k - Pr_k); 
%% ── STEP 3: State-Dependent Volumes (gamma) ─────────────────────────────
% Calculate instantaneous fluid stiffness
V_A = V_0 + A_c * x1;
V_B = V_0 - A_c * x1;

% Prevent volumes from dropping below zero geometrically
V_A = max(1e-6, V_A);
V_B = max(1e-6, V_B);

gamma_A = beta / V_A;
gamma_B = beta / V_B;

%% ── STEP 4: Build SDC Matrices (A6 and f6) ──────────────────────────────
% A6: Internal couplings and linear leakages + Disturbance Dynamics
A6 = [0,  1,               0,                 0,                0,          0;
      0,  a22,             A_c/M,            -A_c/M,            1/M,        0;
      0, -gamma_A*A_c,    -gamma_A*C_t,       gamma_A*C_t,      0,          gamma_A;
      0,  gamma_B*A_c,     gamma_B*C_t,      -gamma_B*C_t,      0,         -gamma_B;
      0,  0,               0,                 0,               -alpha_Fd,   0;
      0,  0,               0,                 0,                0,         -alpha_Qd];

% f6: External physical forces, flow inputs, and hard nonlinearities
f6 = [0;
      0;
      gamma_A * Q1;
      gamma_B * Q2; 
      0;
      0];

% Forward Euler Discrete Integration
A_d6 = I6 + dt * A6;   

%% ── STEP 5: Scale Transform ──────────────────────────────────────────────
A_d6_sc = (SC6 * SCI6') .* A_d6;   
x_sc    = SC6 .* x_hat;
f_sc    = SC6 .* f6;

%% ── STEP 6: Kalman Predict ───────────────────────────────────────────────
x_pred_sc = A_d6_sc * x_sc + dt * f_sc; 

P_pred = A_d6_sc * P_k * A_d6_sc' + Q_d6;
P_pred = 0.5*(P_pred + P_pred'); 

%% ── STEP 7: Innovation & Kalman Gain ─────────────────────────────────────
z_sc   = [SC6(1)*y_k(1); SC6(3)*y_k(2); SC6(4)*y_k(3)];
innov  = z_sc - C_sc6 * x_pred_sc;
S6     = C_sc6 * P_pred * C_sc6' + R_m6;
S6     = 0.5 * (S6 + S6');

if rcond(S6) < 1e-14
    S6 = S6 + 1e-12 * eye(3);
end

K6    = (P_pred * C_sc6') / S6;
IKH6  = I6 - K6 * C_sc6;
P_k   = IKH6 * P_pred * IKH6' + K6 * R_m6 * K6'; % Joseph Form olarak bilinir. $A P A^T + B R B^T$ y
P_k   = 0.5 * (P_k + P_k');

%% ── STEP 8: Update & Output ──────────────────────────────────────────────
x_hat = SCI6 .* (x_pred_sc + K6 * innov);

% Hard physical clamp on updated pressures
x_hat(3) = max(0, min(Ps_k, x_hat(3)));
x_hat(4) = max(0, min(Ps_k, x_hat(4)));

% Map to outputs
x_hat_out = x_hat;
Fd_est    = x_hat(5);
Qd_est    = x_hat(6);

end

== matlab function NonLinModelMracScaled/Plant/Subsystem1/MATLAB Function ==
  data: Q1 output; Q2 output; x input; Ps input; Pr input; P1 input; P2 input; K input; k input; QR output
function [Q1, Q2, QR] = fcn(x, Ps, Pr, P1, P2, K, k)
    % x0 parametresini girişten kaldırdık, içeride asimetrik tanımlayacağız.
    
    % --- ASİMETRİK SIZINTI AYARLARI ---
    % Hedef: P_null = 70 bar (Ps=210 bar iken)
    % Bu dengeyi sağlamak için Return tarafı açıklığı daha büyük olmalı.

    % --- GÜNCELLENMİŞ ASİMETRİK SIZINTI AYARLARI ---
    % Hedef: Ps=200 bar, Pr=4.5 bar iken yaklaşık 70-75 bar denge basıncı
    % $$x_{0S} \cdot \sqrt{130} = x_{0R} \cdot \sqrt{70}$$ --> Ortalamaları
    % da bulunan x0 olacak.

    % Ortalama x0 = 0.53e-3 idi. Bunu asimetrik dağıtıyoruz:
    % x0_S = 0.47e-3;  % Supply tarafı (0.47 mA)
    % x0_R = 0.64e-3;  % Return tarafı (0.64 mA)
    
    x0_S = 0.46e-3 ;  % Supply tarafı (0.46 mA) --> bunu editledim
    x0_R = 0.64e-3 ;  % Return tarafı (0.64 mA)

    % x0_S = 0.53e-3;  % Supply tarafı (0.47 mA)
    % x0_R = 0.53e-3;  % Return tarafı (0.64 mA)

    K_tare = 2.345e-9; 
    
    % Güvenlik (Basınçlar)
    dPs1 = max(0, Ps - P1); dP1r = max(0, P1 - Pr);
    dPs2 = max(0, Ps - P2); dP2r = max(0, P2 - Pr);
    dPsr = max(0, Ps - Pr);

    if x >= 0
        % P_S -> P_1 (Supply Side - Ana Akış) -> x0_S kullan
        Q1_S = K * sqrt(dPs1) * (x0_S + x); 
        
        % P_1 -> P_R (Return Side - Sızıntı) -> x0_R kullan
        Q1_R = K * sqrt(dP1r) * (x0_R^2 / (x0_R + k*x)); 

        % P_S -> P_2 (Supply Side - Sızıntı) -> x0_S kullan
        Q2_S = K * sqrt(dPs2) * (x0_S^2 / (x0_S + k*x)); 
        
        % P_2 -> P_R (Return Side - Ana Akış) -> x0_R kullan
        Q2_R = K * sqrt(dP2r) * (x0_R + x);
    else
        % x < 0 durumu
        % Simetriyi korumak için x negatifken de Supply/Return rollerine göre
        % doğru x0'ı seçmeliyiz.
        
        % P_S -> P_1 (Supply Side - Sızıntı)
        Q1_S = K * sqrt(dPs1) * (x0_S^2 / (x0_S - k*x)); 
        
        % P_1 -> P_R (Return Side - Ana Akış)
        Q1_R = K * sqrt(dP1r) * (x0_R - x); 

        % P_S -> P_2 (Supply Side - Ana Akış)
        Q2_S = K * sqrt(dPs2) * (x0_S - x); 
        
        % P_2 -> P_R (Return Side - Sızıntı)
        Q2_R = K * sqrt(dP2r) * (x0_R^2 / (x0_R - k*x)); 
    end

    Q1 = Q1_S - Q1_R;
    Q2 = Q2_S - Q2_R;
    QR = Q1_R + (Q2_R) + K_tare * sqrt(dPsr); 
end

== matlab function NonLinModelMracScaled/Plant/Cylinder_Dynamics/Subsystem1/MATLAB Function1 ==
  data: x input; F_end output; x_dot input; xmin input; xmax input; k_end input; v_lock input
function F_end = endstop_force_simple(x, x_dot, xmin, xmax, k_end, v_lock)
%#codegen
% Very stable end-stop with velocity locking
% Minimal oscillation, solver-friendly

% v_lock : velocity below which motion is considered zero (m/s)
% Typical: 1e-3 … 5e-3

F_end = 0.0;
ccc = 1e6; 
% ---- LOWER STOP ----
if x <= xmin
    % spring force
    F_end = k_end * (xmin - x);

    % velocity lock (kill oscillation)
    if x_dot < v_lock
        F_end = F_end - ccc * x_dot;   % artificial strong damping
    end
end

% ---- UPPER STOP ----
if x >= xmax
    % spring force
    F_end = -k_end * (x - xmax);

    % velocity lock
    if x_dot > -v_lock
        F_end = F_end - ccc * x_dot;
    end
end

== matlab function NonLinModelMracScaled/Plant/Cylinder_Dynamics/Subsystem/Subsystem/MATLAB Function ==
  data: v input; F_statik output
function F_statik = fcn(v)
Fc = 18; 
Fs = 75; 
v_s = 0.016; 
C = 100; 

F_statik = Fc + (Fs - Fc)*exp(-(1*abs(v)./v_s)^2);
F_statik = F_statik * tanh(C*v);

== matlab function NonLinModelMracScaled/Plant/Cylinder_Dynamics/Friction_Simple ==
  data: v input; FF output
function FF = fcn(v)
eps_smooth = 0.1; 

% --- Pozitif Yön (v > 0) ---
kv_p = 20; kc_p = 15; ks_p = 82.9; tau_p = 0.016;

% --- Negatif Yön (v < 0) ---
kv_n = 35; kc_n = 22; ks_n = 75.17; tau_n = 0.016;

% Yumuşatılmış yön fonksiyonu (sign yerine tanh)
% Bu fonksiyon -1 ile 1 arasında yumuşak bir geçiş sağlar
smooth_sign = tanh(v ./ eps_smooth);

% Asimetrik katsayı vektörleri oluşturma
% Hızın yönüne göre katsayıları seçiyoruz
kv = (v >= 0)*kv_p + (v < 0)*kv_n;
kc = (v >= 0)*kc_p + (v < 0)*kc_n;
ks = (v >= 0)*ks_p + (v < 0)*ks_n;
tau = (v >= 0)*tau_p + (v < 0)*tau_n;

% --- Sürtünme Kuvveti Hesaplama ---
% F_viscous + F_coulomb + F_stribeck
FF = (kv .* v) + (kc .* smooth_sign) + (ks .* smooth_sign .* exp(-abs(v./tau)));

== matlab function NonLinModelMracScaled/Plant/Cylinder_Dynamics/Subsystem/Kalman_Jerk_xa ==
  settings: updateMethod=DISCRETE
  data: pos_meas input; v_est output; acc_meas input; dt input; a_est output; j_est output
function [v_est, a_est, j_est] = fcn(pos_meas, acc_meas, dt)
    % KALMAN FİLTRESİ (Jerk Augmented)
    % Durumlar: x = [Pozisyon; Hız; İvme; Jerk]
    
    % Değişkenleri hafızada tutmak için 'persistent' tanımlıyoruz
    persistent x P A H Q R I initialized
    
    % --- BAŞLANGIÇ AYARLARI (Sadece ilk adımda çalışır) ---
    if isempty(initialized)
        % Başlangıç Durumu (İlk ölçüme göre)
        x = [pos_meas; 0; acc_meas; 0]; 
        
        % Başlangıç Belirsizliği
        P = eye(4); 
        
        % Matris Tanımları (Sabitler)
        % 1. Geçiş Matrisi (Fizik: x = x0 + v*dt + 0.5*a*dt^2 + ...)
        A = [1, dt, 0.5*dt^2, (1/6)*dt^3;
             0,  1,       dt,   0.5*dt^2;
             0,  0,        1,         dt;
             0,  0,        0,          1];
         
        % 2. Ölçüm Matrisi (Sadece Pos ve Acc ölçüyoruz)
        H = [1, 0, 0, 0;
             0, 0, 1, 0];
         
        % 3. Gürültü Kovaryansları (TUNING BURADAN)
        sigma_jerk = 2000; % Sistemin vahşiliği (Spike yakalama yeteneği)
        
        % Q (Süreç Gürültüsü)
        Q = diag([dt^6/36, dt^4/4, dt^2, 1]) * sigma_jerk^2;
        
        % R (Ölçüm Gürültüsü) - Sensör güveni
        R_pos = (1e-6)^2;
        R_acc = (0.5)^2;
        R = diag([R_pos, R_acc]);
        
        I = eye(4);
        initialized = 1;
    end
    
    % --- KALMAN DÖNGÜSÜ (Her adımda çalışır) ---
    
    % 1. PREDICT (Öngörü)
    x_pred = A * x;
    P_pred = A * P * A' + Q;
    
    % 2. UPDATE (Düzeltme)
    z = [pos_meas; acc_meas]; % Ölçüm vektörü
    
    y = z - H * x_pred;       % Innovation (Hata)
    S = H * P_pred * H' + R;  % Innovation Covaryans
    K = P_pred * H' / S;      % Kalman Kazancı
    
    x = x_pred + K * y;       % Durum Güncelleme
    P = (I - K * H) * P_pred; % Kovaryans Güncelleme
    
    % 3. ÇIKTI
    v_est = x(2);
    a_est = x(3);
    j_est = x(4);
end

== matlab function NonLinModelMracScaled/Plant/Cylinder_Dynamics/Subsystem/Kalman_Jerk_xPaPb ==
  settings: updateMethod=DISCRETE
  data: j_est output; a_est output; pos_meas input; v_est output; PA input; PB input
function [j_est, a_est, v_est] = fcn(pos_meas, PA, PB)
    % PRESSURE-AIDED JERK ESTIMATOR
    % Girdiler: Pozisyon ve Basınçlar
    % Çıktı: Tertemiz Jerk (j_est)
    
    persistent x P A H Q R I initialized m AA AB
    
    % --- SABİTLER ---
    dt = 0.001;   % Örnekleme Zamanı (Simulink step size ile aynı olmalı)
    
    if isempty(initialized)
        % 1. SİSTEM TANIMLAMALARI
        m  = 3.4;       % Tahmini Hareketli Kütle (kg)
        AA = 2.0106e-04;  % A Odası Alanı (m2)
        AB = 2.0106e-04;  % B Odası Alanı (m2)
        
        % 2. DURUM VEKTÖRÜ: x = [Konum; Hız; İvme; Jerk]
        % (Sürtünme değil, doğrudan kinematiği izliyoruz)
        F_net_start = (PA*AA - PB*AB);
        a_start = F_net_start / m;
        
        x = [pos_meas; 0; a_start; 0];
        P = eye(4);
        I = eye(4);
        
        % 3. GEÇİŞ MATRİSİ (Constant Jerk Model)
        % x(k+1) = x(k) + v*dt + 0.5*a*dt^2 + 1/6*j*dt^3 ...
        A = [1, dt, 0.5*dt^2, (1/6)*dt^3;
             0,  1,       dt,   0.5*dt^2;
             0,  0,        1,         dt;
             0,  0,        0,          1];
         
        % 4. ÖLÇÜM MATRİSİ
        % z1 = Konum (x1)
        % z2 = İvme  (x3) -> Basınçtan türetilmiş "Sanal İvme"
        H = [1, 0, 0, 0;
             0, 0, 1, 0];
         
        % 5. TUNING (AYARLAR)
        % Q: Jerk ne kadar hızlı değişebilir? (Sistemin vahşiliği)
        % Yüksek değer = Zıplamaları anında yakalar (Gecikmesiz).
        sigma_jerk = 100; 
        Q = diag([dt^6/36, dt^4/4, dt^2, 1]) * sigma_jerk^2;
        
        % R: Ölçümlere ne kadar güveniyoruz?
        R_pos = (1e-6)^2; % Konum çok hassas
        R_acc = (2.0)^2;  % Basınçtan gelen ivme "gürültülüdür" (Sürtünme yok sayıldığı için)
                          % Burayı gevşek bırakıyoruz ki Kalman, konum verisiyle
                          % basınç verisini harmanlayıp doğruyu bulsun.
        R = diag([R_pos, R_acc]);
        
        initialized = 1;
    end
    
    % --- 1. SANAL İVME ÖLÇÜMÜ OLUŞTURMA ---
    % Basınç kuvvetini kütleye bölerek "Ham İvme" elde ediyoruz.
    % Not: Bu ivme sürtünmeyi içermez, bu yüzden "gürültülü/hatalı" kabul edilir.
    % Kalman bunu düzeltecek.
    F_hyd = PA * AA - PB * AB;
    a_meas_virtual = F_hyd / m; 
    
    % Ölçüm Vektörü
    z = [pos_meas; a_meas_virtual];
    
    % --- 2. KALMAN PREDICT ---
    x_pred = A * x;
    P_pred = A * P * A' + Q;
    
    % --- 3. KALMAN UPDATE ---
    y = z - H * x_pred;       % Hata (Innovation)
    S = H * P_pred * H' + R;  % Kovaryans
    K = P_pred * H' / S;      % Kazanç (Gain)
    
    x = x_pred + K * y;       % Güncelleme
    P = (I - K * H) * P_pred;
    
    % --- 4. ÇIKTILAR ---
    v_est = x(2);
    a_est = x(3);
    j_est = x(4); % İŞTE ARADIĞIN JERK!
end

== matlab function NonLinModelMracScaled/Plant/Cylinder_Dynamics/Subsystem/Subsystem1/MATLAB Function ==
  data: v input; F_statik output
function F_statik = fcn(v)
Fc = 18; 
Fs = 75; 
v_s = 0.016; 
C = 100; 

F_statik = Fc + (Fs - Fc)*exp(-(1*abs(v)./v_s)^2);
F_statik = F_statik * tanh(C*v);

== matlab function NonLinModelMracScaled/Plant/Cylinder_Dynamics/MATLAB Function1 ==
  data: v input; FF output; a input; j input
function FF = fcn(v,a,j)
% --- Geçiş Yumuşaklığı Parametresi ---
% Bu değer büyüdükçe 0'daki eğim azalır (daha eğimli geçer)
eps_smooth = 0.00223;


% --- Pozitif Yön (v > 0) ---
kv_p = 39.658; Fc_p = 25; Fs_p = 82.9; tau_p = 0.0016;

% --- Negatif Yön (v < 0) ---
kv_n = 38.5; Fc_n = 5; Fs_n = 75.17; tau_n = 0.0016;

% Yumuşatılmış yön fonksiyonu (sign yerine tanh)
% Bu fonksiyon -1 ile 1 arasında yumuşak bir geçiş sağlar
smooth_sign = tanh(v ./ eps_smooth);

% Asimetrik katsayı vektörleri oluşturma
% Hızın yönüne göre katsayıları seçiyoruz
kv = (v >= 0)*kv_p + (v < 0)*kv_n;
Fc = (v >= 0)*Fc_p + (v < 0)*Fc_n;
Fs = (v >= 0)*Fs_p + (v < 0)*Fs_n;
tau = (v >= 0)*tau_p + (v < 0)*tau_n;

F_stribeck = (kv .* v) + (Fc .* smooth_sign) + (Fs .* smooth_sign .* exp(-abs(v./tau)));

K_acc = 1.121235; 
K_jerk = 0.056481; 
kappa_delay = 0; 

FF = F_stribeck + K_acc * a  +  K_jerk*j;
